simulink model "velDutyRespTest"  (R2025a)
settings: Solver=VariableStepAuto  StartTime=0.0  StopTime=4  RelTol=1e-3
InitFcn:
  | addpath('SCADA');
  | initFcn_SCADA;
values from neighbouring files (symbols this model uses):
  pump1Duty = -0.0    (= 0)    [run_velDutyRespTest.m]
  pump2Duty = -0.    (= 0)    [run_velDutyRespTest.m]
undefined symbols (not defined in the file or in its folder): National_Instruments, PCIe
libraries: sldrtlib x5
settings Model: Creator=simmo536  LastModifiedBy=simmo536

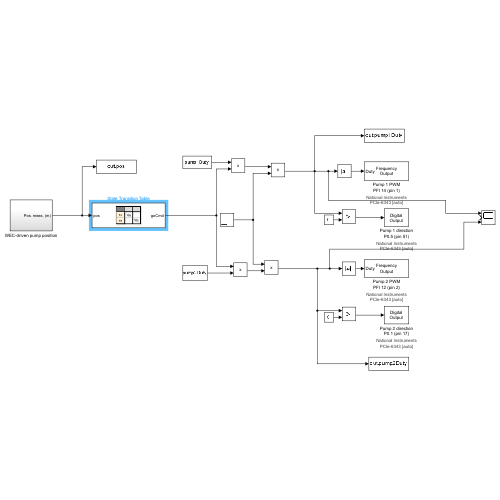
[thumbnail: Simulink's stored preview of the top-level diagram]
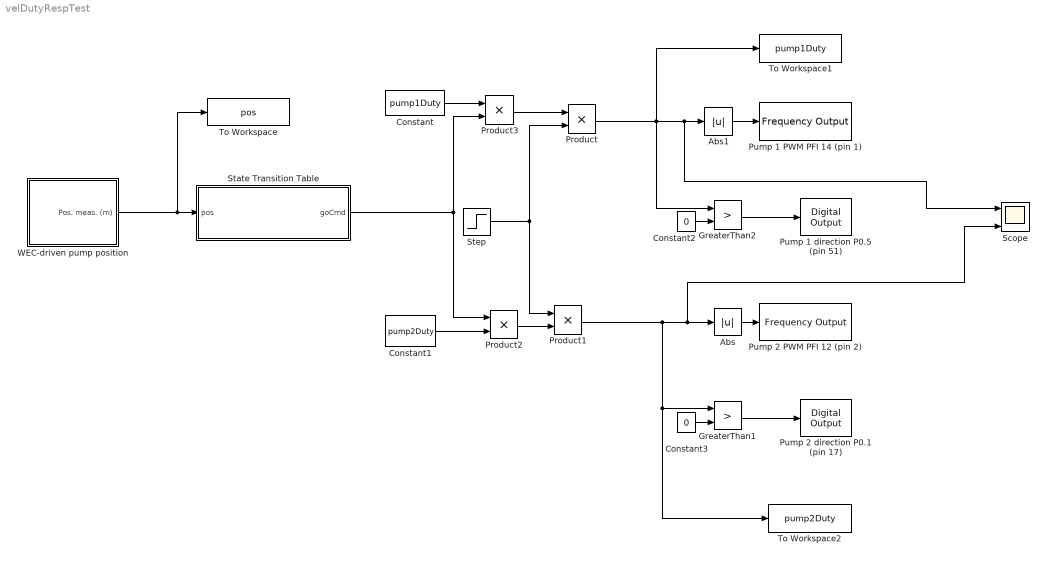
== system velDutyRespTest ==
  Abs : Abs  SaturateOnIntegerOverflow=off
  Abs1 : Abs  SaturateOnIntegerOverflow=off
  Constant : Constant  Value=pump1Duty
  Constant1 : Constant  Value=pump2Duty
  Constant2 : Constant  Value=0
  Constant3 : Constant  Value=0
  GreaterThan1 : RelationalOperator  Operator=>  OutDataTypeStr=boolean  RndMeth=Simplest  InputSameDT=off
  GreaterThan2 : RelationalOperator  Operator=>  OutDataTypeStr=boolean  RndMeth=Simplest  InputSameDT=off
  Product{,1..3} (4 alike) : Product
  Pump 1 PWM PFI 14 (pin 1) : sldrtlib/Frequency Output  SampleTime=0.1  MaxMissedTicks=inf  ShowMissedTicks=off  YieldWhenWaiting=off  DrvName=National_Instruments/PCIe-6343  DrvAddress=4294967295  DrvOptions=[0 4479 48128 3 3 3 3]  Channels=3  FrequencySource=1  Frequency=100  FrequencyFinalValue=[]  DutySource=2  Duty=0  DutyFinalValue=0
      settings: AttributesFormatString=National Instruments\nPCIe-6343 [auto]
  Pump 1 direction P0.5 (pin 51) : sldrtlib/Digital Output  SampleTime=0.1  MaxMissedTicks=10  ShowMissedTicks=off  YieldWhenWaiting=off  DrvName=National_Instruments/PCIe-6343  DrvAddress=4294967295  DrvOptions=[0 4479 48128 3 3 3 3]  Channels=6  BitMode=1  InitialValue=1  FinalValue=1
      settings: AttributesFormatString=National Instruments\nPCIe-6343 [auto]
  Pump 2 PWM PFI 12 (pin 2) : sldrtlib/Frequency Output  SampleTime=0.1  MaxMissedTicks=inf  ShowMissedTicks=off  YieldWhenWaiting=off  DrvName=National_Instruments/PCIe-6343  DrvAddress=4294967295  DrvOptions=[0 4479 48128 3 3 3 3]  Channels=1  FrequencySource=1  Frequency=100  FrequencyFinalValue=[]  DutySource=2  Duty=0  DutyFinalValue=0
      settings: AttributesFormatString=National Instruments\nPCIe-6343 [auto]
  Pump 2 direction P0.1 (pin 17) : sldrtlib/Digital Output  SampleTime=0.1  MaxMissedTicks=10  ShowMissedTicks=off  YieldWhenWaiting=off  DrvName=National_Instruments/PCIe-6343  DrvAddress=4294967295  DrvOptions=[0 4479 48128 3 3 3 3]  Channels=2  BitMode=1  InitialValue=0  FinalValue=0
      settings: AttributesFormatString=National Instruments\nPCIe-6343 [auto]
  Scope : Scope  NumInputPorts=3
      settings: ActiveDisplayYMinimum=-0.452887537993921  ActiveDisplayYMaximum=0.25835866261398177
  State Transition Table : State Transition Table  TreatAsAtomicUnit=on
  Step : Step  Time=0.1  SampleTime=0
  To Workspace : ToWorkspace  VariableName=pos  SaveFormat=Timeseries  SampleTime=-1
  To Workspace1 : ToWorkspace  VariableName=pump1Duty  SaveFormat=Timeseries  SampleTime=-1
  To Workspace2 : ToWorkspace  VariableName=pump2Duty  SaveFormat=Timeseries  SampleTime=-1
  WEC-driven pump position : Subsystem
  wires:
  WEC-driven pump position/1(Pos. meas. (m)) -> To Workspace/1, State Transition Table/1(pos)
  GreaterThan2/1 -> Pump 1 direction P0.5 (pin 51)/1
  GreaterThan1/1 -> Pump 2 direction P0.1 (pin 17)/1
  Constant/1 -> Product3/1
  Step/1 -> Product1/1, Product/2
  Abs/1 -> Pump 2 PWM PFI 12 (pin 2)/1
  Product2/1 -> Product1/2
  Constant1/1 -> Product2/2
  Product3/1 -> Product/1
  State Transition Table/1(goCmd) -> Product3/2, Product2/1
  Abs1/1 -> Pump 1 PWM PFI 14 (pin 1)/1
  Constant3/1 -> GreaterThan1/2
  Product1/1 -> Scope/3, Abs/1, To Workspace2/1, GreaterThan1/1
  Constant2/1 -> GreaterThan2/2
  Product/1 -> GreaterThan2/1, To Workspace1/1, Scope/1, Abs1/1

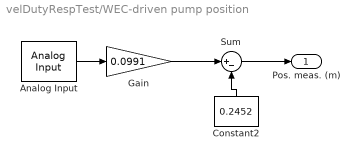
== system velDutyRespTest/WEC-driven pump position ==
  Analog Input : sldrtlib/Analog Input  SampleTime=0.0001  MaxMissedTicks=inf  ShowMissedTicks=off  YieldWhenWaiting=on  DrvName=National_Instruments/PCIe-6343  DrvAddress=4294967295  DrvOptions=[0 4479 48128 3 3 3 3]  Channels=8  RangeMode=1  VoltRange=1  DataType=1
      settings: AttributesFormatString=National Instruments\nPCIe-6343 [auto]
  Constant2 : Constant  Value=0.2452
  Gain : Gain  Gain=0.0991
  Sum : Sum  Inputs=|+-
  Pos. meas. (m) : Outport
  wires:
  Constant2/1 -> Sum/2
  Gain/1 -> Sum/1
  Analog Input/1 -> Gain/1
  Sum/1 -> Pos. meas. (m)/1

== stateflow chart velDutyRespTest/State Transition Table ==
  state init
    entry:
    goCmd=0;
  state idle
    entry:
    goCmd=0;
  state goFromCenterZone
    entry:
    goCmd=1;
  state goFromPosBuffer
    entry:
    goCmd=1;
  state goFromNegBuffer
    entry:
    goCmd=1;
  state stop
    entry:
    goCmd=0;
  state terminal
  (default) -> init
  init -> idle : [true]
  idle -> (junction 118) [order 2] : [pos>=15*0.0254]
  (junction 118) -> (junction 116)
  idle -> (junction 123) [order 3] : [pos<=-7*0.0254]
  (junction 123) -> (junction 121)
  idle -> goFromCenterZone [order 1] : [pos>=-7*0.0254 && pos<=15*0.0254]
  goFromCenterZone -> (junction 109) : [pos<=-7*0.0254 || pos>=15*0.0254]
  (junction 109) -> (junction 126)
  (junction 116) -> goFromPosBuffer
  goFromPosBuffer -> (junction 126) : [pos<=-7*0.0254 || pos>=15*0.0254]
  (junction 126) -> (junction 107)
  (junction 121) -> goFromNegBuffer
  goFromNegBuffer -> stop : [pos<=-8*0.0254 || pos>=7*0.0254]
  (junction 107) -> stop
  stop -> terminal : [true]
  terminal -> (junction 102)
  (junction 102) -> terminal
  data: pos input; goCmd output
